simulink model "sampleModel1953"  (R2023a)
settings: Solver=VariableStepAuto  StartTime=0.0  StopTime=10.0  RelTol=1e-3
libraries: simulink x3, hdlsllib x2
settings Model: Creator=user1  LastModifiedBy=user1

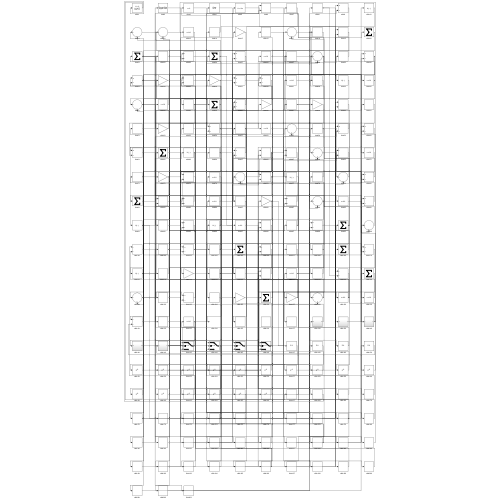
[thumbnail: Simulink's stored preview of the top-level diagram]
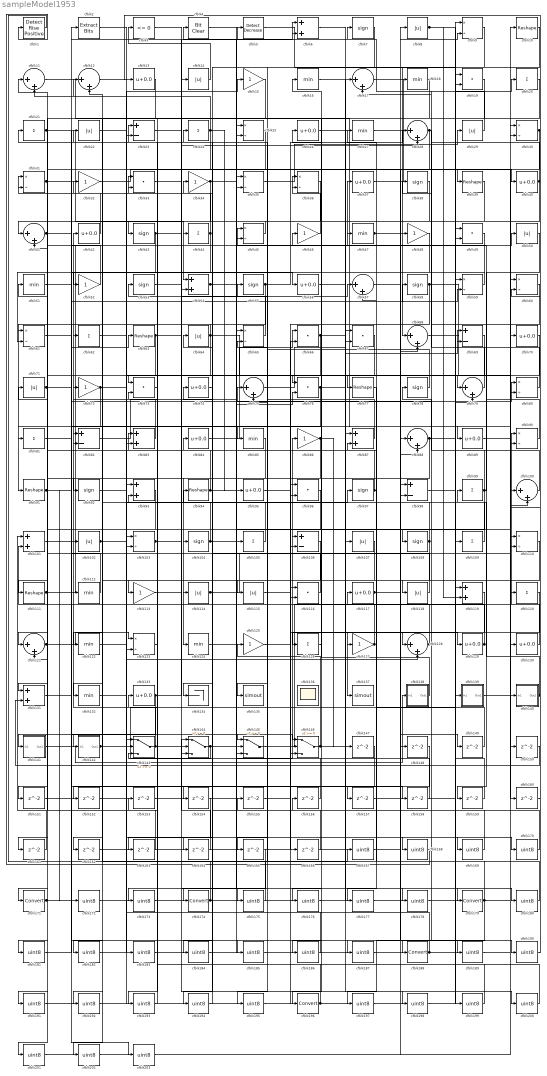
== system sampleModel1953 ==
  cfblk1 : hdlsllib/Logic and Bit Operations/Detect Rise Positive  vinit=0  OutDataTypeStr=boolean
  cfblk{10,39,63,77,91,94,111} (7 alike) : Reshape
  cfblk{11..12,17,28,41,57,68,75,79,88,100,121,128} (13 alike) : Sum  Inputs=|++
  cfblk{6,54,83,87,93,101,119,131} (8 alike) : Sum
  cfblk{8,14,22,29,50,64,71,102,107,114..115,118} (12 alike) : Abs  SaturateOnIntegerOverflow=off
  cfblk{9,25,30..31,35..36,45,59..61,65,80,90,103,110,123} (16 alike) : Product  Inputs=*/  RndMeth=Zero  SaturateOnIntegerOverflow=on
  cfblk{7,38,43,53,55,58,78,92,97,104,108} (11 alike) : Signum
  cfblk{20..21,24,44,62,81,99,105,109,120,126} (11 alike) : Sum  Inputs=+
  cfblk{23,69,82,98,106} (5 alike) : Sum  Inputs=+-
  cfblk{16,18,27,47,51,85,112,122,124,132} (10 alike) : MinMax
  cfblk{15,32,34,46,48,52,72,86,113,125,127} (11 alike) : Gain
  cfblk{19,33,49,66..67,73,76,96,116} (9 alike) : DotProduct  OutDataTypeStr=Inherit: Inherit via internal rule
  cfblk{13,26,37,40,42,56,70,74,84,89,95,117,129..130,133} (15 alike) : Bias  Bias=0.0  SaturateOnIntegerOverflow=off
  cfblk134 : Terminator
  cfblk135 : ToWorkspace  VariableName=simout  SaveFormat=Timeseries  SampleTime=-1
  cfblk136 : Scope
      settings: Floating=on
  cfblk137 : ToWorkspace  VariableName=simout  SaveFormat=Timeseries  SampleTime=-1
  cfblk138 : Subsystem
      settings: LibrarySourceBlock=|
      | hdlsllib/Ports &
      | Subsystems/Subsystem
  cfblk139 : Subsystem
      settings: LibrarySourceBlock=|
      | hdlsllib/Ports &
      | Subsystems/Subsystem
  cfblk140 : Subsystem
      settings: LibrarySourceBlock=|
      | hdlsllib/Ports &
      | Subsystems/Subsystem
  cfblk141 : Subsystem
      settings: LibrarySourceBlock=|
      | hdlsllib/Ports &
      | Subsystems/Subsystem
  cfblk142 : Subsystem
      settings: LibrarySourceBlock=|
      | hdlsllib/Ports &
      | Subsystems/Subsystem
  cfblk{143..146} (4 alike) : Switch  SaturateOnIntegerOverflow=off  InputSameDT=off
  cfblk{147..166} (20 alike) : Delay  SampleTime=1
  cfblk{167..170,172..173,175..178,180..187,189..195,197..203} (32 alike) : DataTypeConversion  OutDataTypeStr=uint8  SaturateOnIntegerOverflow=off  RndMeth=Floor
  cfblk{171,174,179,188,196} (5 alike) : DataTypeConversion  SaturateOnIntegerOverflow=off  RndMeth=Floor
  cfblk2 : simulink/Logic and Bit Operations/Extract Bits  bitsToExtract=Upper half  numBits=8  bitIdxRange=[0 7]  outScalingMode=Preserve fixed-point scaling
      settings: LibrarySourceBlock=|
      | hdlsllib/Logic and Bit
      | Operations/Extract Bits
  cfblk3 : hdlsllib/Logic and Bit Operations/Compare To Zero  relop=<=  OutDataTypeStr=boolean
  cfblk4 : simulink/Logic and Bit Operations/Bit Clear  iBit=0
      settings: LibrarySourceBlock=|
      | hdlsllib/Logic and Bit
      | Operations/Bit Clear
  cfblk5 : simulink/Logic and Bit Operations/Detect Decrease  vinit=0.0  OutDataTypeStr=boolean
      settings: LibrarySourceBlock=|
      | hdlsllib/Logic and Bit
      | Operations/Detect
      | Decrease
  wires:
  cfblk143/1 -> cfblk42/1, cfblk198/1
  cfblk40/1 -> cfblk4/1, cfblk83/2
  cfblk142/1(Out1) -> cfblk86/1, cfblk109/1, cfblk97/1, cfblk128/2
  cfblk85/1 -> cfblk124/1
  cfblk88/1 -> cfblk20/1, cfblk161/1
  cfblk123/1 -> cfblk23/1
  cfblk37/1 -> cfblk40/1
  cfblk130/1 -> cfblk90/1
  cfblk11/1 -> cfblk108/1
  cfblk49/1 -> cfblk196/1
  cfblk67/1 -> cfblk171/1
  cfblk108/1 -> cfblk114/1, cfblk12/2
  cfblk20/1 -> cfblk73/1
  cfblk24/1 -> cfblk121/1, cfblk95/1, cfblk11/2
  cfblk9/1 -> cfblk68/1
  cfblk32/1 -> cfblk39/1
  cfblk92/1 -> cfblk15/1
  cfblk126/1 -> cfblk26/1
  cfblk86/1 -> cfblk144/2, cfblk147/1
  cfblk42/1 -> cfblk31/1
  cfblk111/1 -> cfblk37/1, cfblk146/3
  cfblk141/1(Out1) -> cfblk138/1(In1)
  cfblk59/1 -> cfblk52/1
  cfblk87/1 -> cfblk21/1
  cfblk118/1 -> cfblk16/1
  cfblk121/1 -> cfblk123/1, cfblk110/1
  cfblk112/1 -> cfblk51/1
  cfblk129/1 -> cfblk62/1, cfblk112/1
  cfblk29/1 -> cfblk7/1
  cfblk90/1 -> cfblk45/1
  cfblk34/1 -> cfblk92/1, cfblk146/1
  cfblk103/1 -> cfblk157/1, cfblk158/1
  cfblk43/1 -> cfblk61/2, cfblk5/1, cfblk175/1
  cfblk91/1 -> cfblk63/1, cfblk172/1
  cfblk145/1 -> cfblk30/1
  cfblk80/1 -> cfblk38/1
  cfblk107/1 -> cfblk134/1
  cfblk69/1 -> cfblk118/1
  cfblk119/1 -> cfblk137/1
  cfblk51/1 -> cfblk50/1
  cfblk96/1 -> cfblk104/1
  cfblk21/1 -> cfblk54/1, cfblk90/2, cfblk54/2
  cfblk36/1 -> cfblk131/1
  cfblk4/1 -> cfblk65/1
  cfblk14/1 -> cfblk3/1
  cfblk66/1 -> cfblk132/1, cfblk59/2, cfblk75/2, cfblk135/1
  cfblk55/1 -> cfblk91/1, cfblk28/1
  cfblk100/1 -> cfblk78/1
  cfblk62/1 -> cfblk103/1
  cfblk27/1 -> cfblk130/1
  cfblk133/1 -> cfblk57/1, cfblk201/1
  cfblk38/1 -> cfblk43/1
  cfblk61/1 -> cfblk89/1
  cfblk30/1 -> cfblk122/1, cfblk115/1
  cfblk65/1 -> cfblk33/1
  cfblk102/1 -> cfblk142/1(In1), cfblk144/3
  cfblk74/1 -> cfblk174/1
  cfblk23/1 -> cfblk79/1
  cfblk116/1 -> cfblk34/1
  cfblk84/1 -> cfblk66/1
  cfblk124/1 -> cfblk105/1
  cfblk75/1 -> cfblk17/1
  cfblk104/1 -> cfblk22/1, cfblk178/1
  cfblk146/1 -> cfblk107/1, cfblk65/2
  cfblk76/1 -> cfblk81/1, cfblk36/2, cfblk69/2
  cfblk127/1 -> cfblk101/2, cfblk45/2
  cfblk15/1 -> cfblk141/1(In1)
  cfblk140/1(Out1) -> cfblk13/1, cfblk99/1
  cfblk139/1(Out1) -> cfblk30/2
  cfblk114/1 -> cfblk87/1, cfblk76/2
  cfblk99/1 -> cfblk75/1, cfblk121/2, cfblk69/1
  cfblk82/1 -> cfblk6/1
  cfblk53/1 -> cfblk179/1
  cfblk138/1(Out1) -> cfblk106/1
  cfblk2/1 -> cfblk56/1
  cfblk5/1 -> cfblk119/1
  cfblk73/1 -> cfblk113/1
  cfblk128/1 -> cfblk126/1, cfblk82/2
  cfblk64/1 -> cfblk111/1, cfblk61/1, cfblk88/2
  cfblk78/1 -> cfblk55/1
  cfblk63/1 -> cfblk123/2, cfblk143/2, cfblk28/2
  cfblk54/1 -> cfblk46/1, cfblk76/1
  cfblk79/1 -> cfblk17/2
  cfblk26/1 -> cfblk88/1
  cfblk3/1 -> cfblk85/1
  cfblk44/1 -> cfblk32/1, cfblk162/1
  cfblk45/1 -> cfblk41/1
  cfblk8/1 -> cfblk139/1(In1), cfblk119/2
  cfblk97/1 -> cfblk71/1, cfblk57/2
  cfblk94/1 -> cfblk83/1, cfblk110/2
  cfblk117/1 -> cfblk9/2, cfblk190/1
  cfblk72/1 -> cfblk77/1, cfblk151/1
  cfblk60/1 -> cfblk188/1
  cfblk131/1 -> cfblk80/1
  cfblk35/1 -> cfblk29/1
  cfblk41/1 -> cfblk2/1, cfblk154/1
  cfblk47/1 -> cfblk8/1, cfblk80/2
  cfblk31/1 -> cfblk44/1, cfblk203/1
  cfblk12/1 -> cfblk145/1
  cfblk33/1 -> cfblk14/1
  cfblk58/1 -> cfblk140/1(In1), cfblk146/2
  cfblk28/1 -> cfblk103/2, cfblk128/1, cfblk145/3
  cfblk144/1 -> cfblk35/1, cfblk143/3
  cfblk71/1 -> cfblk41/2, cfblk58/1
  cfblk46/1 -> cfblk36/1
  cfblk6/1 -> cfblk129/1
  cfblk115/1 -> cfblk127/1
  cfblk52/1 -> cfblk11/1
  cfblk17/1 -> cfblk70/1
  cfblk105/1 -> cfblk82/1
  cfblk81/1 -> cfblk6/2
  cfblk83/1 -> cfblk72/1
  cfblk13/1 -> cfblk23/2
  cfblk68/1 -> cfblk100/2
  cfblk109/1 -> cfblk47/1
  cfblk57/1 -> cfblk149/1
  cfblk149/1 -> cfblk87/2
  cfblk150/1 -> cfblk131/2
  cfblk151/1 -> cfblk106/2
  cfblk110/1 -> cfblk152/1
  cfblk152/1 -> cfblk35/2
  cfblk153/1 -> cfblk66/2
  cfblk156/1 -> cfblk116/1
  cfblk157/1 -> cfblk9/1
  cfblk158/1 -> cfblk145/2
  cfblk50/1 -> cfblk159/1
  cfblk159/1 -> cfblk59/1
  cfblk89/1 -> cfblk160/1
  cfblk160/1 -> cfblk100/1
  cfblk161/1 -> cfblk101/1
  cfblk162/1 -> cfblk68/2
  cfblk39/1 -> cfblk163/1
  cfblk163/1 -> cfblk31/2
  cfblk10/1 -> cfblk164/1
  cfblk164/1 -> cfblk144/1
  cfblk70/1 -> cfblk165/1
  cfblk95/1 -> cfblk166/1
  cfblk166/1 -> cfblk24/1
  cfblk1/1 -> cfblk167/1
  cfblk167/1 -> cfblk117/1
  cfblk155/1 -> cfblk168/1
  cfblk168/1 -> cfblk1/1
  cfblk125/1 -> cfblk169/1
  cfblk169/1 -> cfblk156/1
  cfblk122/1 -> cfblk170/1
  cfblk170/1 -> cfblk125/1
  cfblk171/1 -> cfblk79/2, cfblk116/2
  cfblk172/1 -> cfblk67/1
  cfblk154/1 -> cfblk173/1
  cfblk173/1 -> cfblk67/2
  cfblk174/1 -> cfblk12/1, cfblk73/2
  cfblk175/1 -> cfblk74/1
  cfblk19/1 -> cfblk176/1
  cfblk176/1 -> cfblk150/1
  cfblk77/1 -> cfblk177/1
  cfblk177/1 -> cfblk19/1
  cfblk178/1 -> cfblk19/2
  cfblk179/1 -> cfblk155/1, cfblk27/1, cfblk197/1
  cfblk113/1 -> cfblk180/1
  cfblk180/1 -> cfblk53/1
  cfblk25/1 -> cfblk181/1
  cfblk181/1 -> cfblk102/1
  cfblk147/1 -> cfblk182/1
  cfblk182/1 -> cfblk25/1
  cfblk22/1 -> cfblk183/1
  cfblk183/1 -> cfblk25/2
  cfblk148/1 -> cfblk184/1
  cfblk184/1 -> cfblk96/2
  cfblk132/1 -> cfblk185/1
  cfblk185/1 -> cfblk148/1
  cfblk120/1 -> cfblk186/1
  cfblk186/1 -> cfblk64/1
  cfblk101/1 -> cfblk187/1
  cfblk187/1 -> cfblk120/1
  cfblk188/1 -> cfblk143/1, cfblk33/2
  cfblk16/1 -> cfblk189/1
  cfblk189/1 -> cfblk60/1
  cfblk190/1 -> cfblk60/2
  cfblk93/1 -> cfblk191/1
  cfblk191/1 -> cfblk96/1
  cfblk106/1 -> cfblk192/1
  cfblk192/1 -> cfblk93/1
  cfblk165/1 -> cfblk193/1
  cfblk193/1 -> cfblk93/2
  cfblk48/1 -> cfblk194/1
  cfblk194/1 -> cfblk84/1
  cfblk7/1 -> cfblk195/1
  cfblk195/1 -> cfblk48/1
  cfblk196/1 -> cfblk153/1, cfblk133/1
  cfblk197/1 -> cfblk49/1
  cfblk198/1 -> cfblk49/2
  cfblk98/1 -> cfblk199/1
  cfblk199/1 -> cfblk94/1
  cfblk56/1 -> cfblk200/1
  cfblk200/1 -> cfblk98/1
  cfblk201/1 -> cfblk98/2
  cfblk18/1 -> cfblk202/1
  cfblk202/1 -> cfblk10/1
  cfblk203/1 -> cfblk18/1

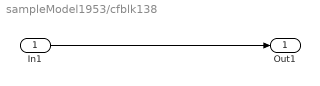
== system sampleModel1953/cfblk138 ==
  In1 : Inport
  Out1 : Outport
  wires:
  In1/1 -> Out1/1

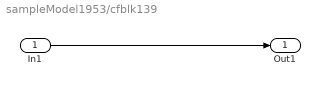
== system sampleModel1953/cfblk139 ==
  In1 : Inport
  Out1 : Outport
  wires:
  In1/1 -> Out1/1

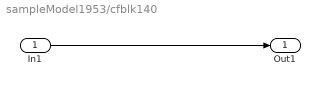
== system sampleModel1953/cfblk140 ==
  In1 : Inport
  Out1 : Outport
  wires:
  In1/1 -> Out1/1

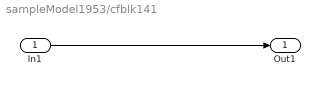
== system sampleModel1953/cfblk141 ==
  In1 : Inport
  Out1 : Outport
  wires:
  In1/1 -> Out1/1

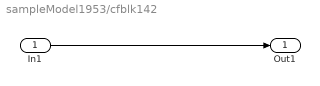
== system sampleModel1953/cfblk142 ==
  In1 : Inport
  Out1 : Outport
  wires:
  In1/1 -> Out1/1
